simulink model "task_2"  (R2021b)
settings: Solver=VariableStepAuto  StartTime=0.0  StopTime=10.0  RelTol=1e-3
libraries: commanapbnd3 x1, dspfdesign x1
settings Model: Creator=aleksejshevcenko  LastModifiedBy=aleksejshevcenko

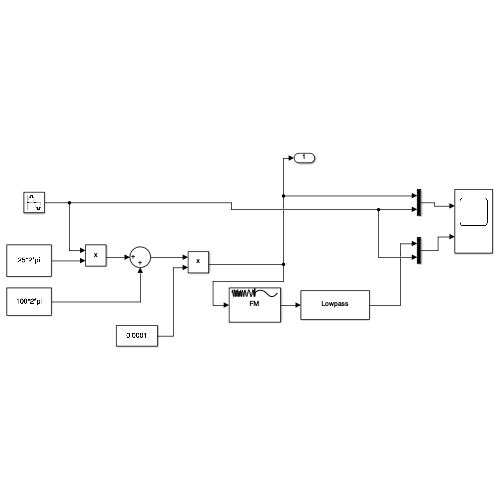
[thumbnail: Simulink's stored preview of the top-level diagram]
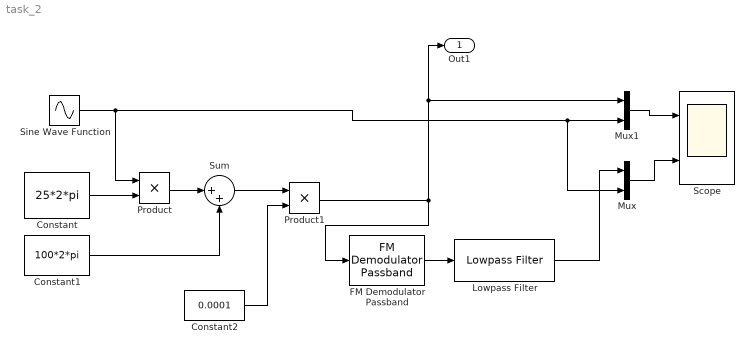
== system task_2 ==
  Constant : Constant  Value=25*2*pi
  Constant1 : Constant  Value=100*2*pi
  Constant2 : Constant  Value=0.0001
  FM Demodulator Passband : commanapbnd3/FM Demodulator Passband  Fc=100  Ph=0  Kc=25  Ho=100
      settings: SourceProductBaseCode=CM
  Lowpass Filter : dspfdesign/Lowpass Filter  FilterType=FIR  DesignForMinimumOrder=on  FilterOrder=50  PassbandFrequency=0.1  StopbandFrequency=100  PassbandRipple=0.1  StopbandAttenuation=80  InheritSampleRate=on  SampleRate=44100  SimulateUsing=Interpreted execution  roundingMode=Floor  coeffsDataTypeStr=fixdt(1,16)
  Mux : Mux  Inputs=2
  Mux1 : Mux  Inputs=2
  Product : Product
  Product1 : Product
  Scope : Scope  NumInputPorts=2
  Sine Wave Function : Sin  Frequency=2*2*pi  SampleTime=0.0001
  Sum : Sum  Inputs=|++
  Out1 : Outport
  wires:
  Mux1/1 -> Scope/1
  Mux/1 -> Scope/2
  Lowpass Filter/1 -> Mux/1
  Sine Wave Function/1 -> Mux/2, Mux1/2, Product/1
  FM Demodulator Passband/1 -> Lowpass Filter/1
  Constant/1 -> Product/2
  Constant1/1 -> Sum/2
  Product/1 -> Sum/1
  Sum/1 -> Product1/1
  Constant2/1 -> Product1/2
  Product1/1 -> Out1/1, Mux1/1, FM Demodulator Passband/1
